simulink model "sim6"  (R2023a)
settings: Solver=VariableStepAuto  StartTime=0  StopTime=300  RelTol=1e-8
settings Model: Creator=vasil  LastModifiedBy=vasil

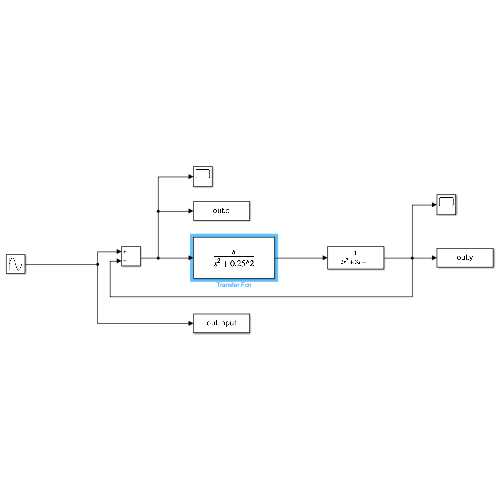
[thumbnail: Simulink's stored preview of the top-level diagram]
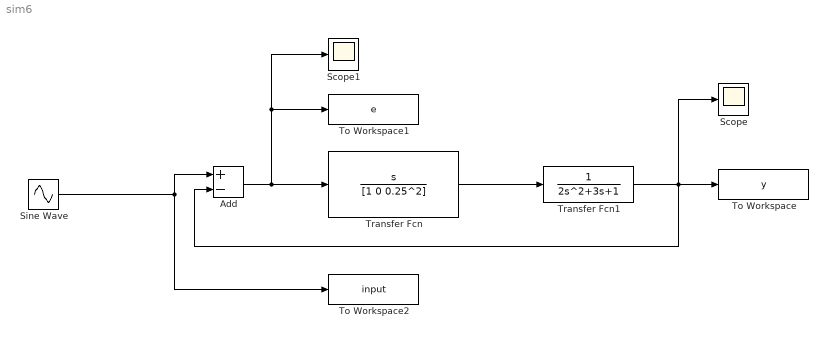
== system sim6 ==
  Add : Sum  Inputs=+-
  Scope : Scope
  Scope1 : Scope
  Sine Wave : Sin  Frequency=0.25  SampleTime=0
  To Workspace : ToWorkspace  VariableName=y  SaveFormat=Timeseries  SampleTime=-1
  To Workspace1 : ToWorkspace  VariableName=e  SaveFormat=Timeseries  SampleTime=-1
  To Workspace2 : ToWorkspace  VariableName=input  SaveFormat=Timeseries  SampleTime=-1
  Transfer Fcn : TransferFcn  Numerator=[1 0]  Denominator=[1 0 0.25^2]
  Transfer Fcn1 : TransferFcn  Denominator=[2 3 1]
  wires:
  Transfer Fcn/1 -> Transfer Fcn1/1
  Add/1 -> Scope1/1, To Workspace1/1, Transfer Fcn/1
  Transfer Fcn1/1 -> Scope/1, To Workspace/1, Add/2
  Sine Wave/1 -> To Workspace2/1, Add/1
